simulink model "integral_control"  (R2016a)
settings: Solver=VariableStepAuto  StartTime=0.0  StopTime=.1  RelTol=1e-4
values from neighbouring files (symbols this model uses):
  K = place(A,B,P)    [calculate_gains.m]
  K1 = K_i(1:2)    [calculate_gains.m]
  K2 = K_i(3)    [calculate_gains.m]
settings Model: Creator=manuel  LastModifiedBy=manuel

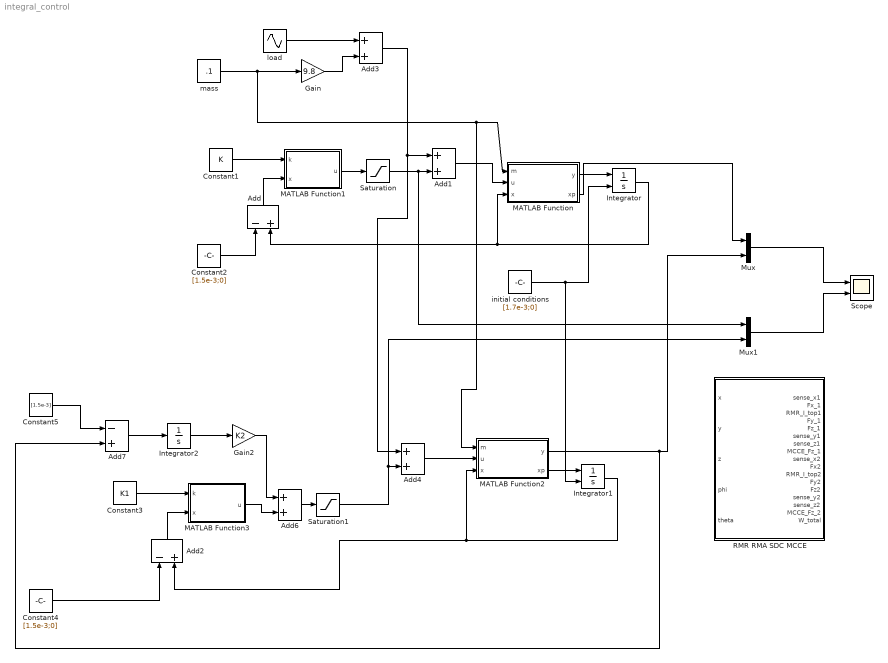
== system integral_control ==
  Add : Sum  Inputs=-+
  Add{1,3..4,6} (4 alike) : Sum
  Add2 : Sum  Inputs=-+
  Add7 : Sum  Inputs=-+
  Constant1 : Constant  Value=K
  Constant2 : Constant  Value=[1.5e-3;0]
  Constant3 : Constant  Value=K1
  Constant4 : Constant  Value=[1.5e-3;0]
  Constant5 : Constant  Value=[1.5e-3]
  Gain : Gain  Gain=9.8
  Gain2 : Gain  Gain=K2
  Integrator : Integrator  InitialConditionSource=external  InitialCondition=[1.6e-3;0]  LimitOutput=on  UpperSaturationLimit=[2e-3;inf]  LowerSaturationLimit=[1e-3;-inf]
  Integrator1 : Integrator  InitialConditionSource=external  InitialCondition=[1.6e-3;0]  LimitOutput=on  UpperSaturationLimit=[2e-3;inf]  LowerSaturationLimit=[1e-3;-inf]
  Integrator2 : Integrator  InitialCondition=[0]  UpperSaturationLimit=[2e-3;inf]  LowerSaturationLimit=[1e-3;-inf]
  MATLAB Function : MATLAB Function  TreatAsAtomicUnit=on
  MATLAB Function1 : MATLAB Function  TreatAsAtomicUnit=on
  MATLAB Function2 : MATLAB Function  TreatAsAtomicUnit=on
  MATLAB Function3 : MATLAB Function  TreatAsAtomicUnit=on
  Mux : Mux  Inputs=2
  Mux1 : Mux  Inputs=2
  RMR RMA SDC MCCE : Subsystem
  Saturation : Saturate  UpperLimit=9.8  LowerLimit=-9.8
  Saturation1 : Saturate  UpperLimit=9.8  LowerLimit=-9.8
  Scope : Scope  NumInputPorts=2
  initial conditions : Constant  Value=[1.7e-3;0]
  load : Sin  Bias=1  Frequency=2*pi*100  SampleTime=0
  mass : Constant  Value=.1
  wires:
  MATLAB Function/2(xp) -> Integrator/1
  Integrator/1 -> MATLAB Function/3(x), Add/2
  MATLAB Function/1(y) -> Mux/1
  Constant1/1 -> MATLAB Function1/1(k)
  Constant2/1 -> Add/1
  Add/1 -> MATLAB Function1/2(x)
  Add1/1 -> MATLAB Function/2(u)
  Gain/1 -> Add3/2
  load/1 -> Add3/1
  Mux/1 -> Scope/1
  Mux1/1 -> Scope/2
  MATLAB Function1/1(u) -> Saturation/1
  Saturation/1 -> Mux1/1, Add1/2
  MATLAB Function2/2(xp) -> Integrator1/1
  Integrator1/1 -> Add2/2, MATLAB Function2/3(x)
  MATLAB Function2/1(y) -> Add7/2, Mux/2
  Constant3/1 -> MATLAB Function3/1(k)
  Constant4/1 -> Add2/1
  Add2/1 -> MATLAB Function3/2(x)
  Add4/1 -> MATLAB Function2/2(u)
  Add3/1 -> Add4/1, Add1/1
  initial conditions/1 -> Integrator1/2, Integrator/2
  Saturation1/1 -> Mux1/2, Add4/2
  Integrator2/1 -> Gain2/1
  Add6/1 -> Saturation1/1
  Gain2/1 -> Add6/1
  MATLAB Function3/1(u) -> Add6/2
  Add7/1 -> Integrator2/1
  Constant5/1 -> Add7/1
  mass/1 -> Gain/1, MATLAB Function2/1(m), MATLAB Function/1(m)

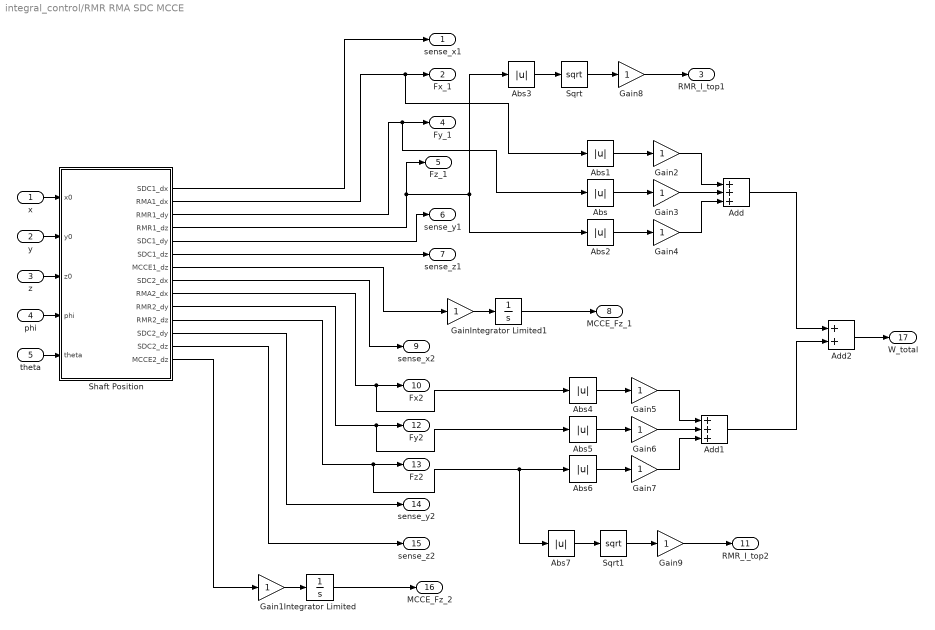
== system integral_control/RMR RMA SDC MCCE ==
  x : Inport
  y : Inport  Port=2
  z : Inport  Port=3
  phi : Inport  Port=4
  theta : Inport  Port=5
  Abs{,1..7} (8 alike) : Abs
  Add : Sum  Inputs=+++
  Add1 : Sum  Inputs=+++
  Add2 : Sum
  Gain{,1..9} (10 alike) : Gain
  Integrator Limited : Integrator  LimitOutput=on  UpperSaturationLimit=1  LowerSaturationLimit=0
  Integrator Limited1 : Integrator  LimitOutput=on  UpperSaturationLimit=1  LowerSaturationLimit=0
  Shaft Position : MATLAB Function  TreatAsAtomicUnit=on
  Sqrt : Sqrt  SaturateOnIntegerOverflow=on
  Sqrt1 : Sqrt  SaturateOnIntegerOverflow=on
  sense_x1 : Outport
  Fx_1 : Outport  Port=2
  RMR_I_top1 : Outport  Port=3
  Fy_1 : Outport  Port=4
  Fz_1 : Outport  Port=5
  sense_y1 : Outport  Port=6
  sense_z1 : Outport  Port=7
  MCCE_Fz_1 : Outport  Port=8
  sense_x2 : Outport  Port=9
  Fx2 : Outport  Port=10
  RMR_I_top2 : Outport  Port=11
  Fy2 : Outport  Port=12
  Fz2 : Outport  Port=13
  sense_y2 : Outport  Port=14
  sense_z2 : Outport  Port=15
  MCCE_Fz_2 : Outport  Port=16
  W_total : Outport  Port=17
  wires:
  y/1 -> Shaft Position/2(y0)
  x/1 -> Shaft Position/1(x0)
  z/1 -> Shaft Position/3(z0)
  phi/1 -> Shaft Position/4(phi)
  theta/1 -> Shaft Position/5(theta)
  Add/1 -> Add2/1
  Shaft Position/1(SDC1_dx) -> sense_x1/1
  Shaft Position/3(RMR1_dy) -> Fy_1/1, Abs/1
  Shaft Position/4(RMR1_dz) -> Fz_1/1, Abs2/1, Abs3/1
  Shaft Position/5(SDC1_dy) -> sense_y1/1
  Shaft Position/6(SDC1_dz) -> sense_z1/1
  Gain/1 -> Integrator Limited1/1
  Shaft Position/7(MCCE1_dz) -> Gain/1
  Integrator Limited1/1 -> MCCE_Fz_1/1
  Shaft Position/12(SDC2_dy) -> sense_y2/1
  Shaft Position/13(SDC2_dz) -> sense_z2/1
  Shaft Position/14(MCCE2_dz) -> Gain1/1
  Gain3/1 -> Add/2
  Gain2/1 -> Add/1
  Gain4/1 -> Add/3
  Shaft Position/2(RMA1_dx) -> Abs1/1, Fx_1/1
  Add1/1 -> Add2/2
  Shaft Position/9(RMA2_dx) -> Abs4/1, Fx2/1
  Shaft Position/10(RMR2_dy) -> Abs5/1, Fy2/1
  Gain6/1 -> Add1/2
  Gain5/1 -> Add1/1
  Gain7/1 -> Add1/3
  Shaft Position/8(SDC2_dx) -> sense_x2/1
  Shaft Position/11(RMR2_dz) -> Abs7/1, Abs6/1, Fz2/1
  Add2/1 -> W_total/1
  Sqrt/1 -> Gain8/1
  Gain8/1 -> RMR_I_top1/1
  Abs1/1 -> Gain2/1
  Abs/1 -> Gain3/1
  Abs2/1 -> Gain4/1
  Abs3/1 -> Sqrt/1
  Abs4/1 -> Gain5/1
  Abs5/1 -> Gain6/1
  Abs6/1 -> Gain7/1
  Sqrt1/1 -> Gain9/1
  Gain9/1 -> RMR_I_top2/1
  Abs7/1 -> Sqrt1/1
  Gain1/1 -> Integrator Limited/1
  Integrator Limited/1 -> MCCE_Fz_2/1

== matlab function integral_control/MATLAB Function1 ==
  data: k input; x input; u output
function u = fcn(k,x)
%#codegen

u = -k'*x;

== matlab function integral_control/MATLAB Function ==
  data: m input; u input; x input; y output; xp output
function [y,xp] = mass_model(m,u,x)
%#codegen
A = [0 1
     0 0];
B = [0;
     1/m];
C = [1 0];

xp = A*x + B*u;
y = C*x;

== matlab function integral_control/MATLAB Function2 ==
  data: m input; u input; x input; y output; xp output
function [y,xp] = mass_model(m,u,x)
%#codegen
A = [0 1
     0 0];
B = [0;
     1/m];
C = [1 0];

xp = A*x + B*u;
y = C*x;

== matlab function integral_control/MATLAB Function3 ==
  data: k input; x input; u output
function u = fcn(k,x)
%#codegen

u = -k'*x;

== matlab function integral_control/RMR RMA SDC MCCE/Shaft Position ==
  data: x0 input; SDC1_dx output; y0 input; z0 input; phi input; theta input; RMA1_dx output; RMR1_dy output; RMR1_dz output; SDC1_dy output; SDC1_dz output; MCCE1_dz output; SDC2_dx output; RMA2_dx output; RMR2_dy output; RMR2_dz output; SDC2_dy output; SDC2_dz output; MCCE2_dz output
function [SDC1_dx, RMA1_dx, RMR1_dy, RMR1_dz, SDC1_dy, SDC1_dz, MCCE1_dz, SDC2_dx, RMA2_dx, RMR2_dy, RMR2_dz, SDC2_dy, SDC2_dz, MCCE2_dz] = fcn(x0,y0,z0,phi,theta)
%#codegen
[m,R_r,R_a,I_p,I_0] = system_parameters();

x1 = x(1);
x2 = x(2);
x3 = x(3);
x4 = x(4);
x5 = x(5);
x6 = x(6);
x7 = x(7);
x8 = x(8);
x9 = x(9);
x10 = x(10);

u1 = u(1);
u2 = u(2);
u3 = u(3);
u4 = u(4);
u5 = u(5);

xp = [
	x4;
	x5;
	x6;
	(Fd_x + u5)/m;
	(Fd_y + u1 + u3)/m;
	(Fd_z - (49*m)/5 + u2 + u4)/m;
	x9;
	x10/cos(x8);
	-(R_r*(u2*cos(x8) + u1*sin(x7)*sin(x8)) - Md_y - R_r*(u4*cos(x8) + u3*sin(x7)*sin(x8)) + I_p*ws*x10 + R_a*abs(u5)*cos(x7)*sin(x8))/I_0;
	(Md_z + R_r*u1*cos(x7) - R_r*u3*cos(x7) - R_a*abs(u5)*sin(x7) + I_p*ws*x9)/I_0;
];

y = [
	x1;
	x2 + R_r*cos(x8)*sin(x7);
	x3 - R_r*sin(x8);
	x2 - R_r*cos(x8)*sin(x7);
	x3 + R_r*sin(x8);
];
